simulink model "mod3_counter"  (R2025b)
settings: Solver=VariableStepAuto  StartTime=0.0  StopTime=10.0  RelTol=1e-3
libraries: simulink_extras x3
settings Model: Creator=Johan  LastModifiedBy=Johan

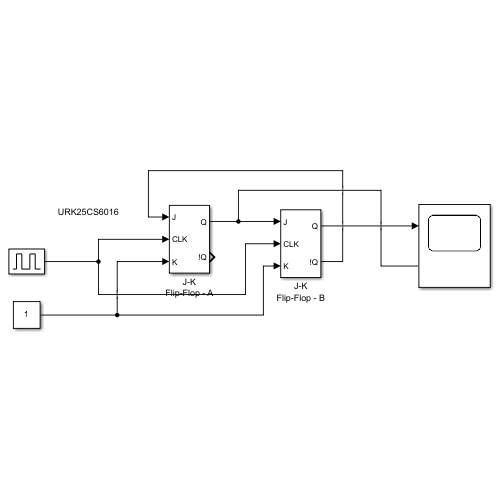
[thumbnail: Simulink's stored preview of the top-level diagram]
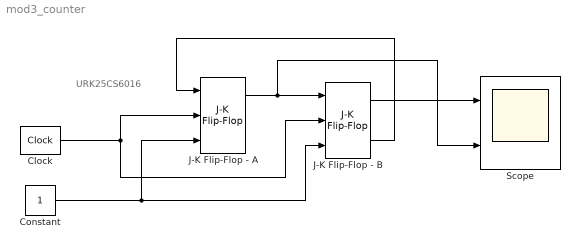
== system mod3_counter ==
  note: URK25CS6016
  Clock : simulink_extras/Flip Flops/Clock  period=2
  Constant : Constant  OutDataTypeStr=boolean
  J-K Flip-Flop - A : simulink_extras/Flip Flops/J-K Flip-Flop  initial_condition=0
  J-K Flip-Flop - B : simulink_extras/Flip Flops/J-K Flip-Flop  initial_condition=0
  Scope : Scope  NumInputPorts=2
      settings: ActiveDisplayYMinimum=-0.12499999999999997  ActiveDisplayYMaximum=1.125
  wires:
  Constant/1 -> J-K Flip-Flop - B/3, J-K Flip-Flop - A/3
  Clock/1 -> J-K Flip-Flop - B/2, J-K Flip-Flop - A/2
  J-K Flip-Flop - B/2 -> J-K Flip-Flop - A/1
  J-K Flip-Flop - A/1 -> Scope/2, J-K Flip-Flop - B/1
  J-K Flip-Flop - B/1 -> Scope/1
